simulink model "tracking1"  (R2019a)
settings: Solver=FixedStepAuto  StartTime=0.0  StopTime=10  FixedStep=0.01  RelTol=1e-3
settings Model: Creator=Dong  LastModifiedBy=Dong

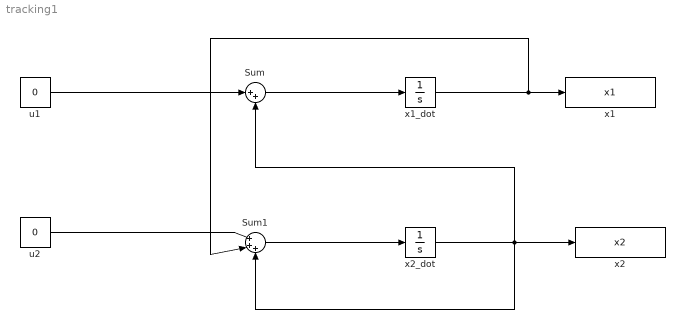
== system tracking1 ==
  Sum : Sum  Inputs=|++
  Sum1 : Sum  Inputs=|+++
  u1 : Constant  Value=0
  u2 : Constant  Value=0
  x1 : ToWorkspace  VariableName=x1  SampleTime=-1
      settings: Save2DSignal=2-D array (concatenate along first dimension)
  x1_dot : Integrator  InitialCondition=1
  x2 : ToWorkspace  VariableName=x2  SampleTime=-1
      settings: Save2DSignal=2-D array (concatenate along first dimension)
  x2_dot : Integrator  InitialCondition=1
  wires:
  x1_dot/1 -> x1/1, Sum1/2
  x2_dot/1 -> x2/1, Sum1/3, Sum/2
  Sum/1 -> x1_dot/1
  Sum1/1 -> x2_dot/1
  u2/1 -> Sum1/1
  u1/1 -> Sum/1
